simulink model "scalar_testing_simulink"  (R2024a)
settings: Solver=FixedStepAuto  StartTime=0.0  StopTime=time_test(end)  FixedStep=ST  RelTol=1e-3
values from neighbouring files (symbols this model uses):
  c_trained = c(end, :)    [scalar_testing_init.m]
  delta = 1.2*u_amplitude/(n_nodes/2)    (= 0.072)    [scalar_training_init.m]
  n_nodes = 50    [scalar_training_init.m]
  ST = 1    [scalar_training_init.m]
settings Model: Creator=gabri  LastModifiedBy=gabri

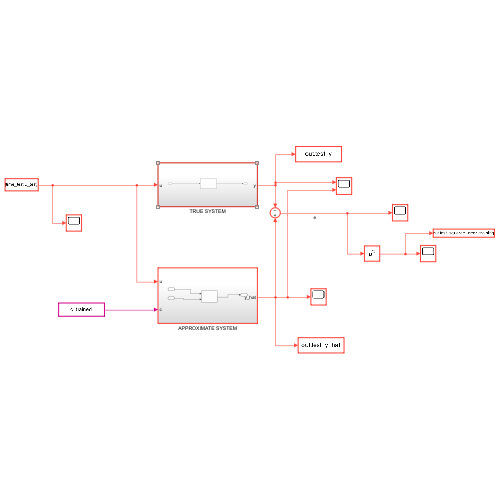
[thumbnail: Simulink's stored preview of the top-level diagram]
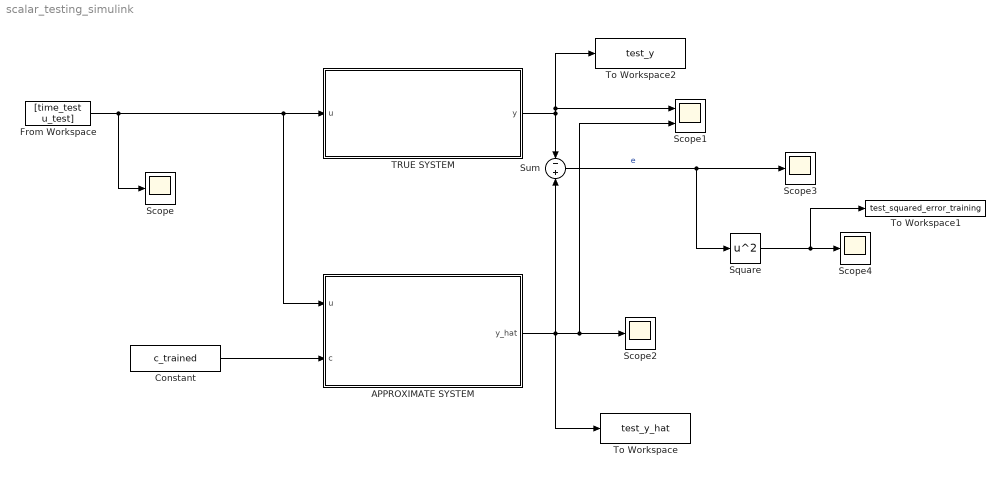
== system scalar_testing_simulink ==
  APPROXIMATE SYSTEM : Subsystem
  Constant : Constant  Value=c_trained
  From Workspace : FromWorkspace  VariableName=[time_test u_test]  SampleTime=ST
  Scope{,2..4} (4 alike) : Scope
  Scope1 : Scope  NumInputPorts=2
  Square : Math  Operator=square
  Sum : Sum  Inputs=-|+
  TRUE SYSTEM : Subsystem
  To Workspace : ToWorkspace  VariableName=test_y_hat  SaveFormat=Timeseries  SampleTime=-1
  To Workspace1 : ToWorkspace  VariableName=test_squared_error_training  SaveFormat=Timeseries  SampleTime=-1
  To Workspace2 : ToWorkspace  VariableName=test_y  SaveFormat=Timeseries  SampleTime=-1
  wires:
  From Workspace/1 -> APPROXIMATE SYSTEM/1(u), TRUE SYSTEM/1(u), Scope/1
  TRUE SYSTEM/1(y) -> To Workspace2/1, Scope1/1, Sum/1
  Sum/1 -> Square/1, Scope3/1  "e"
  Square/1 -> To Workspace1/1, Scope4/1
  Constant/1 -> APPROXIMATE SYSTEM/2(c)
  APPROXIMATE SYSTEM/1(y_hat) -> To Workspace/1, Sum/2, Scope1/2, Scope2/1

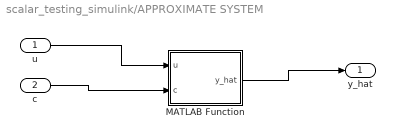
== system scalar_testing_simulink/APPROXIMATE SYSTEM ==
  u : Inport
  c : Inport  Port=2
  MATLAB Function : MATLAB Function  TreatAsAtomicUnit=on
  y_hat : Outport
  wires:
  u/1 -> MATLAB Function/1(u)
  MATLAB Function/1(y_hat) -> y_hat/1
  c/1 -> MATLAB Function/2(c)

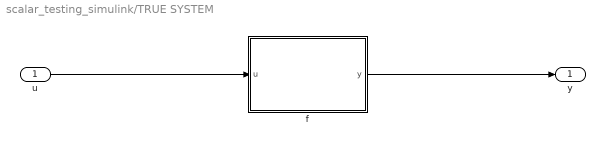
== system scalar_testing_simulink/TRUE SYSTEM ==
  u : Inport
  f : MATLAB Function  TreatAsAtomicUnit=on
  y : Outport
  wires:
  u/1 -> f/1(u)
  f/1(y) -> y/1

== matlab function scalar_testing_simulink/APPROXIMATE SYSTEM/MATLAB Function ==
  data: u input; y_hat output; c input; delta parameter; n_nodes parameter
function y_hat = f_hat(u, c, delta, n_nodes)

y_hat_temp = 0;

shift = ceil(n_nodes/2);

for i = 1:length(c)
    k = i-shift;
    y_hat_temp = y_hat_temp + c(i)*grf(u, k, delta);
end

y_hat = y_hat_temp;

== matlab function scalar_testing_simulink/TRUE SYSTEM/f ==
  data: u input; y output
function y = fcn(u)

y = true_system(u);
